simulink model "P1_ecuaciones_diferenciales_simulink"  (R2023a)
settings: Solver=ode23  StartTime=0.0  StopTime=20  RelTol=1e-3
undefined symbols (not defined in the file): g, l1, l2, m1, m2
settings Model: Creator=karen  LastModifiedBy=karen

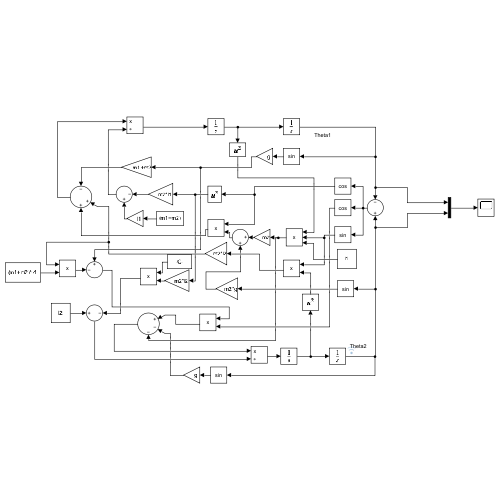
[thumbnail: Simulink's stored preview of the top-level diagram]
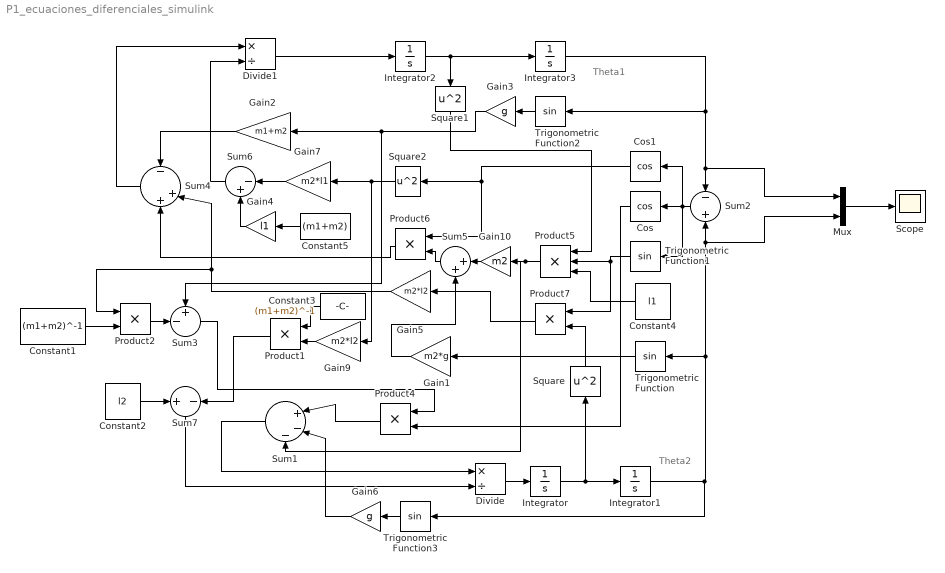
== system P1_ecuaciones_diferenciales_simulink ==
  note: Theta1
  note: Theta2
  Constant1 : Constant  Value=(m1+m2)^-1
  Constant2 : Constant  Value=l2
  Constant3 : Constant  Value=(m1+m2)^-1
  Constant4 : Constant  Value=l1
  Constant5 : Constant  Value=(m1+m2)
  Cos : Trigonometry  Operator=cos
  Cos1 : Trigonometry  Operator=cos
  Divide : Product  Inputs=*/
  Divide1 : Product  Inputs=*/
  Gain1 : Gain  Gain=m2*g
  Gain10 : Gain  Gain=m2
  Gain2 : Gain  Gain=m1+m2
  Gain3 : Gain  Gain=g
  Gain4 : Gain  Gain=l1
  Gain5 : Gain  Gain=m2*l2
  Gain6 : Gain  Gain=g
  Gain7 : Gain  Gain=m2*l1
  Gain9 : Gain  Gain=m2*l2
  Integrator : Integrator  InitialCondition=0.61086
  Integrator1 : Integrator
  Integrator2 : Integrator
  Integrator3 : Integrator
  Mux : Mux  Inputs=2
  Product{1..2,4,6..7} (5 alike) : Product
  Product5 : Product  Inputs=3
  Scope : Scope
  Square : Math  Operator=square
  Square1 : Math  Operator=square
  Square2 : Math  Operator=square
  Sum1 : Sum  Inputs=|+--
  Sum2 : Sum  Inputs=-+
  Sum3 : Sum  Inputs=+-|
  Sum4 : Sum  Inputs=-|++
  Sum5 : Sum  Inputs=|++
  Sum6 : Sum  Inputs=|-+
  Sum7 : Sum  Inputs=+-
  Trigonometric Function{,1..3} (4 alike) : Trigonometry
  wires:
  Integrator3/1 -> Trigonometric Function2/1, Sum2/1, Mux/1
  Sum2/1 -> Cos1/1, Trigonometric Function1/1, Cos/1
  Divide1/1 -> Integrator2/1
  Integrator2/1 -> Integrator3/1, Square1/1
  Trigonometric Function/1 -> Gain1/1
  Gain5/1 -> Sum4/2, Product2/1
  Product4/1 -> Sum1/1
  Mux/1 -> Scope/1
  Trigonometric Function1/1 -> Product7/1, Product5/2
  Square/1 -> Product7/2
  Sum4/1 -> Divide1/1
  Cos1/1 -> Square2/1, Product6/1
  Square1/1 -> Product5/1
  Product7/1 -> Gain5/1
  Cos/1 -> Product4/2
  Divide/1 -> Integrator/1
  Integrator1/1 -> Trigonometric Function3/1, Mux/2, Sum2/2, Trigonometric Function/1
  Sum1/1 -> Divide/1
  Integrator/1 -> Square/1, Integrator1/1
  Trigonometric Function2/1 -> Gain3/1
  Constant3/1 -> Product1/1
  Square2/1 -> Gain9/1, Gain7/1
  Gain7/1 -> Sum6/1
  Gain4/1 -> Sum6/2
  Sum6/1 -> Divide1/2
  Gain3/1 -> Gain2/1, Sum3/1
  Gain2/1 -> Sum4/1
  Constant4/1 -> Product5/3
  Product5/1 -> Gain10/1, Sum1/3
  Product6/1 -> Sum4/3
  Gain1/1 -> Sum5/2
  Sum5/1 -> Product6/2
  Gain9/1 -> Product1/2
  Sum7/1 -> Divide/2
  Product1/1 -> Sum7/2
  Constant2/1 -> Sum7/1
  Constant1/1 -> Product2/2
  Product2/1 -> Sum3/2
  Sum3/1 -> Product4/1
  Trigonometric Function3/1 -> Gain6/1
  Gain6/1 -> Sum1/2
  Gain10/1 -> Sum5/1
  Constant5/1 -> Gain4/1
